simulink library "pmm"  (R2021b)
settings: Solver=VariableStepAuto  StartTime=0.0  StopTime=10.0  RelTol=1e-3
undefined symbols (not defined in the file or in its folder): ENUM_ACMAINRLYSTS_OPEN, ENUM_ACPRECHRGRLYSTS_OPEN, ENUM_B2VRLYSTA_OPEN, ENUM_BMSHVSTS_HVOPEN, ENUM_BRAKEPEDAL_RELEASED, ENUM_CACRLYDEM_CLOSE, ENUM_CACRLYSTS_OPEN, ENUM_CHRGFAULT_ACRLYFAIL, ENUM_CHRGFAULT_BCUHVFAIL, ENUM_CHRGFAULT_BCUNEGFAIL, ENUM_CHRGFAULT_BCUTIMEOUT, ENUM_CHRGFAULT_DCDCENABLE, ENUM_CHRGFAULT_DCDCRLYFAIL, ENUM_CHRGFAULT_HVILFAIL, ENUM_CHRGFAULT_PDUHVFAIL, ENUM_CHRGFAULT_RLYCHKFAIL, ENUM_DCDCEACPCURLYSTA_CLOSED, ENUM_DCDCEACPCURLYSTA_FAILTOCLOSE, ENUM_DCDCEACPCURLYSTA_OPEN, ENUM_DCDCEACPCURLYSTA_WELDED, ENUM_DCDCENABLESTS_READY, ENUM_DCDCRLYSTS_OPEN, ENUM_EHPSRLYDEM_CLOSE, ENUM_EHPSRLYSTS_OPEN, ENUM_FOGRLYENCMD_DISABLE, ENUM_GEARACTUALPOSN_D, ENUM_HVPWROFFREQ_POWEROFF, ENUM_KEYSTATUS_OFF, ENUM_KEYSTATUS_ON, ENUM_KEYSTATUS_START, ENUM_LOWBATTVOLTAGE_NORMAL, ENUM_LOWBATTVOLTAGE_POWERDOWN, ENUM_LOWBATTVOLTAGE_POWERUP, ENUM_MCUHVLOOP_POWEROFF, ENUM_MCUHVLOOPSTS_OPEN, ENUM_MCUMAINRLYSTS_OPEN, ENUM_MCUPRECHRGRLYSTS_OPEN, ENUM_PDFAULT_ACRLYOPEN, ENUM_PDFAULT_BCUDISABLE, ENUM_PDFAULT_DCDCDISABLE, ENUM_PDFAULT_DCDCRLYOPEN, ENUM_PDFAULT_EACDISABLE, ENUM_PDFAULT_EACRLYOPEN, ENUM_PDFAULT_EHPSDISABLE, ENUM_PDFAULT_EHPSRLYOPEN, ENUM_PDFAULT_MCUDISABLE, ENUM_PDFAULT_MCUDISCHRG, ENUM_PDFAULT_MCURLYOPEN, ENUM_PEUSELFCHKSTS_NOFAULT, ENUM_PLUGINSTS_NOPLUGIN, ENUM_PLUGINSTS_PLUGIN, ENUM_PMMMODE_DRIVE, ENUM_PMMMODE_LVBATCHRG, ENUM_PUSTATE_DCDCENABLE, ENUM_PUSTATE_EACPRESCHECK, ENUM_PUSTATE_EHPSENABLE, ENUM_PUSTATE_MCUENABLE, ENUM_PUSTATE_PDUMCURLYCLOSED, ENUM_PUSTATE_POWERUPFAIL, ENUM_TARGETGEAR_REVERSE ... (+126)
libraries: hcu_lib x45, simulink x5, ddm x1, dsc x1
(part 5 of 7)

== system pmm/PMM/PowerModeManagement/PMM State Change Configuration/PMM Initialize to PowerUp State ==
  note: [(VPMM_HVSelfChkCompleted4PU_flg
      | && VPSA_Keystatus_enum == ENUM_KEYSTATUS_START
      | && VINP_DCChrgConnectSts_enum == ENUM_PLUGINSTS_NOPLUGIN)
      |
      | || (!VSCP_LVchrgSvrMode_flg
      | && VPMM_LVChrgPreActFinished_flg
      | && VINP_ParkBrakeSW_flg
      | && VINP_B2VSOC_pct > KPMM_LVChrgEnHVSOC_pct)
      |
      | && (!VPMM_HVILEmergencyStop_flg)]
  VPSA_Keystatus_enum : Inport
  VINP_DCChrgConnectSts_enum : Inport  Port=2
  VPMM_HVILEmergencyStop_flg : Inport  Port=3
  VDMM_ProhibitPowerUp_flg : Inport  Port=4
  VSCP_LVchrgSvrMode_flg : Inport  Port=5
  VPMM_LVChrgPreActFinished_flg : Inport  Port=6
  VINP_ParkBrakeSW_flg : Inport  Port=7
  VINP_B2VSOC_pct : Inport  Port=8
  AND : Logic  Inputs=4  AllPortsSameDT=off  OutDataTypeStr=boolean
  AND1 : Logic  Inputs=5  AllPortsSameDT=off  OutDataTypeStr=boolean
  Constant2 : Constant  Value=ENUM_KEYSTATUS_START
  Constant3 : Constant  Value=ENUM_PLUGINSTS_NOPLUGIN
  Equal : RelationalOperator  Operator===  OutDataTypeStr=boolean  RndMeth=Simplest
  Equal1 : RelationalOperator  Operator===  OutDataTypeStr=boolean  RndMeth=Simplest
  NOT{,1..3} (4 alike) : Logic  Operator=NOT  AllPortsSameDT=off  OutDataTypeStr=boolean
  OR : Logic  Operator=OR  AllPortsSameDT=off  OutDataTypeStr=boolean
  Relay : Relay  OnSwitchValue=KPMM_LVChrgEnHVSOC_pct  OffSwitchValue=KPMM_LVChrgDisHVSOC_pct  OnOutputValue=TRUE  OffOutputValue=FALSE  OutDataTypeStr=boolean
  VPMM_Initialize2PowerUp_flg : Outport
  VPMM_LVChrgInit2PowerUp_flg : Outport  Port=2
  wires:
  NOT1/1 -> AND/4
  [VDMM_ProhibitPowerUp_flg] -> NOT1/1
  [VPSA_Keystatus_enum] -> Equal/1
  Constant2/1 -> Equal/2
  [VPMM_HVILEmergencyStop_flg] -> NOT/1
  VINP_DCChrgConnectSts_enum/1 -> [VINP_DCChrgConnectSts_enum]
  VPMM_HVILEmergencyStop_flg/1 -> [VPMM_HVILEmergencyStop_flg]
  VPSA_Keystatus_enum/1 -> [VPSA_Keystatus_enum]
  [VINP_DCChrgConnectSts_enum] -> Equal1/1
  Constant3/1 -> Equal1/2
  Equal/1 -> AND/1
  Equal1/1 -> AND/2
  NOT/1 -> AND/3
  VDMM_ProhibitPowerUp_flg/1 -> [VDMM_ProhibitPowerUp_flg]
  AND/1 -> OR/1
  OR/1 -> VPMM_Initialize2PowerUp_flg/1  "VPMM_Initialize2PowerUp_flg"
  NOT2/1 -> AND1/1
  [VSCP_LVchrgSvrMode_flg] -> NOT2/1
  [VPMM_LVChrgPreActFinished_flg] -> AND1/2
  [VINP_ParkBrakeSW_flg] -> AND1/3
  [VINP_B2VSOC_pct] -> Relay/1
  Relay/1 -> AND1/4
  AND1/1 -> OR/2, VPMM_LVChrgInit2PowerUp_flg/1  "VPMM_LVChrgInit2PowerUp_flg"
  VSCP_LVchrgSvrMode_flg/1 -> [VSCP_LVchrgSvrMode_flg]
  VPMM_LVChrgPreActFinished_flg/1 -> [VPMM_LVChrgPreActFinished_flg]
  VINP_ParkBrakeSW_flg/1 -> [VINP_ParkBrakeSW_flg]
  VINP_B2VSOC_pct/1 -> [VINP_B2VSOC_pct]
  NOT3/1 -> AND1/5
  [VPMM_HVILEmergencyStop_flg] -> NOT3/1

== system pmm/PMM/PowerModeManagement/PMM State Change Configuration/PMM PowerUp to PowerDown State ==
  note: [VPSA_Keystatus_enum == ENUM_KEYSTATUS_OFF || VPSA_EmergencyShutDown_flg ||
      | VPMM_HVILEmergencyStop_flg ||
      | VPMM_LostCom_flg ||
      | VPMM_RCIncorrect_flg ||
      | VDMM_VCUPowerVolHigh_flg ||
      | VDMM_VCUPowerVolLow_flg ||...
      | VDMM_WireFailure_flg]
  VPSA_Keystatus_enum : Inport
  VPSA_EmergencyShutDown_flg : Inport  Port=2
  VPMM_HVILEmergencyStop_flg : Inport  Port=3
  VPMM_LostCom_flg : Inport  Port=4
  VPMM_RCIncorrect_flg : Inport  Port=5
  VDMM_DCTVCUPowerVolHigh_flg : Inport  Port=6
  VDMM_DTCVCUPowerVolLow_flg : Inport  Port=7
  VDMM_DTCHVILWireFailure_flg : Inport  Port=8
  VDMM_NoFeedBack_flg : Inport  Port=9
  VDMM_WireFailure_flg : Inport  Port=10
  VPMM_LVChrgPreActFinished_flg : Inport  Port=11
  VPMM_PowerUpState_enum : Inport  Port=12
  VINP_B2VSOC_pct : Inport  Port=13
  VINP_ParkBrakeSW_flg : Inport  Port=14
  AND : Logic  AllPortsSameDT=off  OutDataTypeStr=boolean
  Constant : Constant  Value=ENUM_PUSTATE_POWERUPFAIL
  Constant2 : Constant  Value=ENUM_KEYSTATUS_OFF
  Equal : RelationalOperator  Operator===  OutDataTypeStr=boolean  RndMeth=Simplest
  Equal1 : RelationalOperator  Operator===  OutDataTypeStr=boolean  RndMeth=Simplest
  NOT : Logic  Operator=NOT  AllPortsSameDT=off  OutDataTypeStr=boolean
  NOT1 : Logic  Operator=NOT  AllPortsSameDT=off  OutDataTypeStr=boolean
  OR : Logic  Operator=OR  Inputs=11  AllPortsSameDT=off  OutDataTypeStr=boolean
  OR1 : Logic  Operator=OR  Inputs=3  AllPortsSameDT=off  OutDataTypeStr=boolean
  Relay : Relay  OnSwitchValue=KPMM_LVChrgEnHVSOC_pct  OffSwitchValue=KPMM_LVChrgDisHVSOC_pct  OnOutputValue=TRUE  OffOutputValue=FALSE  OutDataTypeStr=boolean
  VPMM_PowerUp2PowerDown_flg : Outport
  wires:
  VPMM_LostCom_flg/1 -> [VPMM_LostCom_flg]
  VPSA_Keystatus_enum/1 -> [VPSA_Keystatus_enum]
  [VPMM_HVILEmergencyStop_flg] -> OR/3
  VPSA_EmergencyShutDown_flg/1 -> [VPSA_EmergencyShutDown_flg]
  [VPMM_LostCom_flg] -> OR/4
  Constant2/1 -> Equal/2
  [VPSA_EmergencyShutDown_flg] -> OR/2
  Equal/1 -> OR/1
  [VPSA_Keystatus_enum] -> Equal/1
  VPMM_HVILEmergencyStop_flg/1 -> [VPMM_HVILEmergencyStop_flg]
  OR/1 -> VPMM_PowerUp2PowerDown_flg/1  "VPMM_PowerUp2PowerDown_flg"
  [VPMM_RCIncorrect_flg] -> OR/5
  VPMM_RCIncorrect_flg/1 -> [VPMM_RCIncorrect_flg]
  VDMM_DCTVCUPowerVolHigh_flg/1 -> [VDMM_DTCVCUPowerVolHigh_flg]
  VDMM_DTCVCUPowerVolLow_flg/1 -> [VDMM_DTCVCUPowerVolLow_flg]
  [VDMM_DTCVCUPowerVolHigh_flg] -> OR/6
  [VDMM_DTCVCUPowerVolLow_flg] -> OR/7
  VDMM_DTCHVILWireFailure_flg/1 -> [VDMM_DTCHVILWireFailure_flg]
  [VDMM_DTCHVILWireFailure_flg] -> OR/8
  VDMM_NoFeedBack_flg/1 -> [VDMM_NoFeedBack_flg]
  [VDMM_NoFeedBack_flg] -> OR/9
  VDMM_WireFailure_flg/1 -> [VDMM_WireFailure_flg]
  [VDMM_WireFailure_flg] -> OR/10
  VPMM_LVChrgPreActFinished_flg/1 -> [VPMM_LVChrgPreActFinished_flg]
  VPMM_PowerUpState_enum/1 -> [VPMM_PowerUpState_enum]
  [VPMM_PowerUpState_enum] -> Equal1/1
  Constant/1 -> Equal1/2
  [VPMM_LVChrgPreActFinished_flg] -> AND/1
  AND/1 -> OR/11
  Equal1/1 -> OR1/1
  [VINP_B2VSOC_pct] -> Relay/1
  NOT/1 -> OR1/3
  [VINP_ParkBrakeSW_flg] -> NOT/1
  OR1/1 -> AND/2
  VINP_B2VSOC_pct/1 -> [VINP_B2VSOC_pct]
  VINP_ParkBrakeSW_flg/1 -> [VINP_ParkBrakeSW_flg]
  Relay/1 -> NOT1/1
  NOT1/1 -> OR1/2

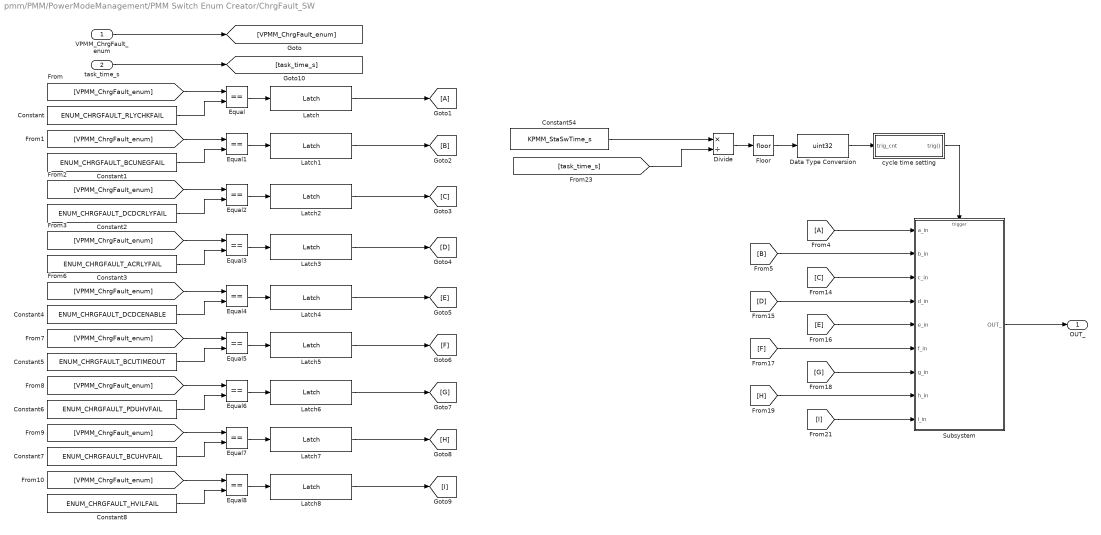
== system pmm/PMM/PowerModeManagement/PMM Switch Enum Creator/ChrgFault_SW ==
  VPMM_ChrgFault_enum : Inport
  task_time_s : Inport  Port=2
  Constant : Constant  Value=ENUM_CHRGFAULT_RLYCHKFAIL
  Constant1 : Constant  Value=ENUM_CHRGFAULT_BCUNEGFAIL
  Constant2 : Constant  Value=ENUM_CHRGFAULT_DCDCRLYFAIL
  Constant3 : Constant  Value=ENUM_CHRGFAULT_ACRLYFAIL
  Constant4 : Constant  Value=ENUM_CHRGFAULT_DCDCENABLE
  Constant5 : Constant  Value=ENUM_CHRGFAULT_BCUTIMEOUT
  Constant54 : Constant  Value=KPMM_StaSwTime_s
  Constant6 : Constant  Value=ENUM_CHRGFAULT_PDUHVFAIL
  Constant7 : Constant  Value=ENUM_CHRGFAULT_BCUHVFAIL
  Constant8 : Constant  Value=ENUM_CHRGFAULT_HVILFAIL
  Data Type Conversion : DataTypeConversion  OutDataTypeStr=uint32
  Divide : Product  Inputs=*/
  Equal{,1..8} (9 alike) : RelationalOperator  Operator===  OutDataTypeStr=boolean  RndMeth=Simplest
  Floor : Rounding
  Latch{,1..8} (9 alike) : hcu_lib/Basic_Blocks/Latch
      settings: SourceProductName=HCU Relative Block Library
  Subsystem : Subsystem
  cycle time setting : Stateflow chart  TreatAsAtomicUnit=on
  OUT_ : Outport
  wires:
  Constant54/1 -> Divide/1
  Divide/1 -> Floor/1
  [task_time_s] -> Divide/2
  Floor/1 -> Data Type Conversion/1
  task_time_s/1 -> [task_time_s]
  Subsystem/1(OUT_) -> OUT_/1
  [I] -> Subsystem/9(i_in)
  [H] -> Subsystem/8(h_in)
  [G] -> Subsystem/7(g_in)
  [F] -> Subsystem/6(f_in)
  [E] -> Subsystem/5(e_in)
  [D] -> Subsystem/4(d_in)
  [C] -> Subsystem/3(c_in)
  [B] -> Subsystem/2(b_in)
  [A] -> Subsystem/1(a_in)
  VPMM_ChrgFault_enum/1 -> [VPMM_ChrgFault_enum]
  [VPMM_ChrgFault_enum] -> Equal/1
  Constant/1 -> Equal/2
  Equal/1 -> Latch/1
  Equal1/1 -> Latch1/1
  Constant1/1 -> Equal1/2
  [VPMM_ChrgFault_enum] -> Equal1/1
  [VPMM_ChrgFault_enum] -> Equal2/1
  Constant2/1 -> Equal2/2
  Equal2/1 -> Latch2/1
  Equal3/1 -> Latch3/1
  Constant3/1 -> Equal3/2
  [VPMM_ChrgFault_enum] -> Equal3/1
  [VPMM_ChrgFault_enum] -> Equal4/1
  Constant4/1 -> Equal4/2
  Equal4/1 -> Latch4/1
  Equal5/1 -> Latch5/1
  Constant5/1 -> Equal5/2
  [VPMM_ChrgFault_enum] -> Equal5/1
  [VPMM_ChrgFault_enum] -> Equal6/1
  Constant6/1 -> Equal6/2
  Equal6/1 -> Latch6/1
  Equal7/1 -> Latch7/1
  Constant7/1 -> Equal7/2
  [VPMM_ChrgFault_enum] -> Equal7/1
  [VPMM_ChrgFault_enum] -> Equal8/1
  Constant8/1 -> Equal8/2
  Equal8/1 -> Latch8/1
  Latch/1 -> [A]
  Latch1/1 -> [B]
  Latch2/1 -> [C]
  Latch5/1 -> [F]
  Latch4/1 -> [E]
  Latch3/1 -> [D]
  Latch8/1 -> [I]
  Latch7/1 -> [H]
  Latch6/1 -> [G]
  Data Type Conversion/1 -> cycle time setting/1(trig_cnt)
  cycle time setting/1(trig()) -> Subsystem/Trigger

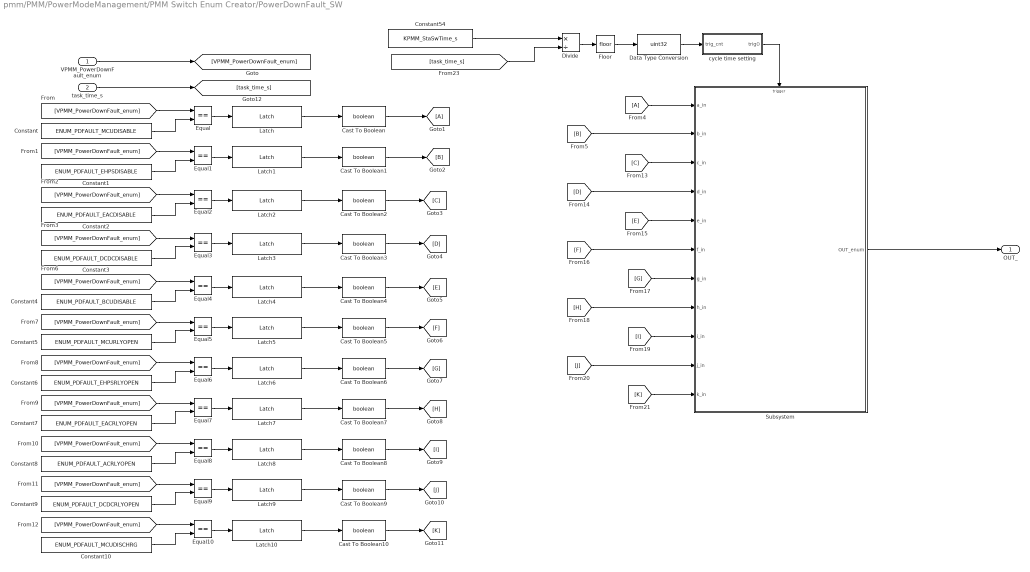
== system pmm/PMM/PowerModeManagement/PMM Switch Enum Creator/PowerDownFault_SW ==
  VPMM_PowerDownFault_enum : Inport
  task_time_s : Inport  Port=2
  Cast To Boolean{,1..10} (11 alike) : DataTypeConversion  OutDataTypeStr=boolean
  Constant : Constant  Value=ENUM_PDFAULT_MCUDISABLE
  Constant1 : Constant  Value=ENUM_PDFAULT_EHPSDISABLE
  Constant10 : Constant  Value=ENUM_PDFAULT_MCUDISCHRG
  Constant2 : Constant  Value=ENUM_PDFAULT_EACDISABLE
  Constant3 : Constant  Value=ENUM_PDFAULT_DCDCDISABLE
  Constant4 : Constant  Value=ENUM_PDFAULT_BCUDISABLE
  Constant5 : Constant  Value=ENUM_PDFAULT_MCURLYOPEN
  Constant54 : Constant  Value=KPMM_StaSwTime_s
  Constant6 : Constant  Value=ENUM_PDFAULT_EHPSRLYOPEN
  Constant7 : Constant  Value=ENUM_PDFAULT_EACRLYOPEN
  Constant8 : Constant  Value=ENUM_PDFAULT_ACRLYOPEN
  Constant9 : Constant  Value=ENUM_PDFAULT_DCDCRLYOPEN
  Data Type Conversion : DataTypeConversion  OutDataTypeStr=uint32
  Divide : Product  Inputs=*/
  Equal{,1..10} (11 alike) : RelationalOperator  Operator===  OutDataTypeStr=boolean  RndMeth=Simplest
  Floor : Rounding
  Latch{,1..10} (11 alike) : hcu_lib/Basic_Blocks/Latch
      settings: SourceProductName=HCU Relative Block Library
  Subsystem : Subsystem
  cycle time setting : Stateflow chart  TreatAsAtomicUnit=on
  OUT_ : Outport
  wires:
  VPMM_PowerDownFault_enum/1 -> [VPMM_PowerDownFault_enum]
  cycle time setting/1(trig()) -> Subsystem/Trigger
  task_time_s/1 -> [task_time_s]
  Constant54/1 -> Divide/1
  Divide/1 -> Floor/1
  [task_time_s] -> Divide/2
  Floor/1 -> Data Type Conversion/1
  [K] -> Subsystem/11(k_in)
  [J] -> Subsystem/10(j_in)
  [I] -> Subsystem/9(i_in)
  [H] -> Subsystem/8(h_in)
  [G] -> Subsystem/7(g_in)
  [F] -> Subsystem/6(f_in)
  [E] -> Subsystem/5(e_in)
  [D] -> Subsystem/4(d_in)
  [C] -> Subsystem/3(c_in)
  [B] -> Subsystem/2(b_in)
  [A] -> Subsystem/1(a_in)
  Subsystem/1(OUT_enum) -> OUT_/1
  Latch6/1 -> Cast To Boolean6/1
  Latch7/1 -> Cast To Boolean7/1
  Latch10/1 -> Cast To Boolean10/1
  Latch9/1 -> Cast To Boolean9/1
  Latch8/1 -> Cast To Boolean8/1
  Latch3/1 -> Cast To Boolean3/1
  Latch4/1 -> Cast To Boolean4/1
  Latch5/1 -> Cast To Boolean5/1
  Latch2/1 -> Cast To Boolean2/1
  Latch1/1 -> Cast To Boolean1/1
  Latch/1 -> Cast To Boolean/1
  Equal10/1 -> Latch10/1
  Constant10/1 -> Equal10/2
  [VPMM_PowerDownFault_enum] -> Equal10/1
  [VPMM_PowerDownFault_enum] -> Equal9/1
  Constant9/1 -> Equal9/2
  Equal9/1 -> Latch9/1
  Equal8/1 -> Latch8/1
  Constant8/1 -> Equal8/2
  [VPMM_PowerDownFault_enum] -> Equal8/1
  [VPMM_PowerDownFault_enum] -> Equal7/1
  Constant7/1 -> Equal7/2
  Equal7/1 -> Latch7/1
  Equal6/1 -> Latch6/1
  Constant6/1 -> Equal6/2
  [VPMM_PowerDownFault_enum] -> Equal6/1
  [VPMM_PowerDownFault_enum] -> Equal5/1
  Constant5/1 -> Equal5/2
  Equal5/1 -> Latch5/1
  Equal4/1 -> Latch4/1
  Constant4/1 -> Equal4/2
  [VPMM_PowerDownFault_enum] -> Equal4/1
  [VPMM_PowerDownFault_enum] -> Equal3/1
  Constant3/1 -> Equal3/2
  Equal3/1 -> Latch3/1
  Equal2/1 -> Latch2/1
  Constant2/1 -> Equal2/2
  [VPMM_PowerDownFault_enum] -> Equal2/1
  [VPMM_PowerDownFault_enum] -> Equal1/1
  Constant1/1 -> Equal1/2
  Equal1/1 -> Latch1/1
  Equal/1 -> Latch/1
  Constant/1 -> Equal/2
  [VPMM_PowerDownFault_enum] -> Equal/1
  Cast To Boolean/1 -> [A]
  Cast To Boolean1/1 -> [B]
  Cast To Boolean2/1 -> [C]
  Cast To Boolean3/1 -> [D]
  Cast To Boolean4/1 -> [E]
  Cast To Boolean5/1 -> [F]
  Cast To Boolean6/1 -> [G]
  Cast To Boolean7/1 -> [H]
  Cast To Boolean8/1 -> [I]
  Cast To Boolean9/1 -> [J]
  Cast To Boolean10/1 -> [K]
  Data Type Conversion/1 -> cycle time setting/1(trig_cnt)

== system pmm/PMM/PowerModeManagement/PMM Switch Enum Creator/PowerUpState_SW ==
  Sys_in : Inport
  a_in : Inport  Port=2
  b_in : Inport  Port=3
  c_in : Inport  Port=4
  d_in : Inport  Port=5
  e_in : Inport  Port=6
  a_enum : Inport  Port=7
  b_enum : Inport  Port=8
  c_enum : Inport  Port=9
  d_enum : Inport  Port=10
  e_enum : Inport  Port=11
  function : TriggerPort  TriggerType=function-call  VariantControl=Variant
  PowerUpState_SW : Stateflow chart  TreatAsAtomicUnit=on
  OUT_enum : Outport
  wires:
  Sys_in/1 -> PowerUpState_SW/1(Sys_in)
  PowerUpState_SW/1(OUT_enum) -> OUT_enum/1
  e_enum/1 -> PowerUpState_SW/11(e_enum)
  d_in/1 -> PowerUpState_SW/5(d_in)
  b_in/1 -> PowerUpState_SW/3(b_in)
  a_enum/1 -> PowerUpState_SW/7(a_enum)
  e_in/1 -> PowerUpState_SW/6(e_in)
  c_in/1 -> PowerUpState_SW/4(c_in)
  a_in/1 -> PowerUpState_SW/2(a_in)
  c_enum/1 -> PowerUpState_SW/9(c_enum)
  d_enum/1 -> PowerUpState_SW/10(d_enum)
  b_enum/1 -> PowerUpState_SW/8(b_enum)

== system pmm/PMM/PowerModeManagement/PMM Flag Creator /HVIL Judgement/Signal reach time counter ==
  signal_in : Inport
  time_step : Inport  Port=2
  time_reach : Inport  Port=3
  cnt_reset : Inport  Port=4
  cnt_max : Inport  Port=5
  cnt_min : Inport  Port=6
  Add : Sum
  Add1 : Sum  Inputs=+-
  Add2 : Sum
  Constant1 : Constant  Value=0
  Constant2 : Constant  OutDataTypeStr=single
  Constant3 : Constant  Value=0  OutDataTypeStr=single
  Logical Operator : Logic  Operator=NOT  AllPortsSameDT=off  OutDataTypeStr=boolean
  Logical Operator1 : Logic  AllPortsSameDT=off  OutDataTypeStr=boolean
  Max : MinMax  Function=max  Inputs=2
  Min : MinMax  Inputs=2
  Relational Operator : RelationalOperator  OutDataTypeStr=boolean  RndMeth=Simplest
  Switch : Switch  Criteria=u2 > Threshold
      settings: AttributesFormatString=%<Criteria>
  Switch1 : Switch  Criteria=u2 > Threshold
      settings: AttributesFormatString=%<Criteria>
  Switch2 : Switch  Criteria=u2 > Threshold
      settings: AttributesFormatString=%<Criteria>
  Unit Delay : UnitDelay  SampleTime=-1  HasFrameUpgradeWarning=on
  Unit Delay1 : UnitDelay  SampleTime=-1  HasFrameUpgradeWarning=on
  Unit Delay2 : UnitDelay  SampleTime=-1  HasFrameUpgradeWarning=on
  cnt_times : Outport
  wires:
  Min/1 -> cnt_times/1
  cnt_max/1 -> Min/2
  Max/1 -> Min/1
  cnt_min/1 -> Max/2
  Constant3/1 -> Switch2/1
  cnt_reset/1 -> Switch2/2
  Switch2/1 -> Unit Delay1/1, Max/1
  Switch/1 -> Switch2/3
  [cont_reset] -> Logical Operator1/2
  signal_in/1 -> Logical Operator1/1
  Logical Operator1/1 -> Switch1/2
  Logical Operator/1 -> [cont_reset]
  [cnt_flg] -> Switch/2
  Unit Delay2/1 -> Logical Operator/1
  Relational Operator/1 -> Unit Delay2/1, [cnt_flg]
  Add2/1 -> Switch/1
  Constant2/1 -> Add2/1
  Unit Delay1/1 -> Add2/2, Switch/3
  time_step/1 -> Add1/2, Add/1
  Unit Delay/1 -> Add/2
  Switch1/1 -> Unit Delay/1, Relational Operator/1
  Add/1 -> Switch1/1
  Constant1/1 -> Switch1/3
  time_reach/1 -> Add1/1
  Add1/1 -> Relational Operator/2

== system pmm/PMM/PowerModeManagement/PMM Flag Creator /HVIL Judgement/Signal reach time counter1 ==
  signal_in : Inport
  time_step : Inport  Port=2
  time_reach : Inport  Port=3
  cnt_reset : Inport  Port=4
  cnt_max : Inport  Port=5
  cnt_min : Inport  Port=6
  Add : Sum
  Add1 : Sum  Inputs=+-
  Add2 : Sum
  Constant1 : Constant  Value=0
  Constant2 : Constant  OutDataTypeStr=single
  Constant3 : Constant  Value=0  OutDataTypeStr=single
  Logical Operator : Logic  Operator=NOT  AllPortsSameDT=off  OutDataTypeStr=boolean
  Logical Operator1 : Logic  AllPortsSameDT=off  OutDataTypeStr=boolean
  Max : MinMax  Function=max  Inputs=2
  Min : MinMax  Inputs=2
  Relational Operator : RelationalOperator  OutDataTypeStr=boolean  RndMeth=Simplest
  Switch : Switch  Criteria=u2 > Threshold
      settings: AttributesFormatString=%<Criteria>
  Switch1 : Switch  Criteria=u2 > Threshold
      settings: AttributesFormatString=%<Criteria>
  Switch2 : Switch  Criteria=u2 > Threshold
      settings: AttributesFormatString=%<Criteria>
  Unit Delay : UnitDelay  SampleTime=-1  HasFrameUpgradeWarning=on
  Unit Delay1 : UnitDelay  SampleTime=-1  HasFrameUpgradeWarning=on
  Unit Delay2 : UnitDelay  SampleTime=-1  HasFrameUpgradeWarning=on
  cnt_times : Outport
  wires:
  Add1/1 -> Relational Operator/2
  time_reach/1 -> Add1/1
  Constant1/1 -> Switch1/3
  Add/1 -> Switch1/1
  Switch1/1 -> Relational Operator/1, Unit Delay/1
  Unit Delay/1 -> Add/2
  time_step/1 -> Add/1, Add1/2
  Unit Delay1/1 -> Switch/3, Add2/2
  Constant2/1 -> Add2/1
  Add2/1 -> Switch/1
  Relational Operator/1 -> [cnt_flg], Unit Delay2/1
  Unit Delay2/1 -> Logical Operator/1
  [cnt_flg] -> Switch/2
  Logical Operator/1 -> [cont_reset]
  Logical Operator1/1 -> Switch1/2
  signal_in/1 -> Logical Operator1/1
  [cont_reset] -> Logical Operator1/2
  Switch/1 -> Switch2/3
  Switch2/1 -> Max/1, Unit Delay1/1
  cnt_reset/1 -> Switch2/2
  Constant3/1 -> Switch2/1
  cnt_min/1 -> Max/2
  Max/1 -> Min/1
  cnt_max/1 -> Min/2
  Min/1 -> cnt_times/1

== system pmm/PMM/PowerModeManagement/PMM Flag Creator /Low Battery Voltage/Long Idle Flasher ==
  task_time_s1 : Inport
  Constant10 : Constant  Value=KPMM_LongIdleBuzzerOFF_s  VectorParams1D=off
  Constant11 : Constant  Value=KPMM_LongIdleBuzzerFlash_cnt  VectorParams1D=off
  Constant12 : Constant  Value=KPMM_LongIdleBuzzerWait_s  VectorParams1D=off
  Constant22 : Constant  Value=KPMM_LongIdleBuzzerON_s  VectorParams1D=off
  Data Type Conversion3 : DataTypeConversion  OutDataTypeStr=boolean
  Reverse Buzzer Flasher : Subsystem
  VPMM_LongIdleBuzzer_flg : Outport
  wires:
  Reverse Buzzer Flasher/1(SigOut) -> Data Type Conversion3/1
  Data Type Conversion3/1 -> VPMM_LongIdleBuzzer_flg/1  "VPMM_LongIdleBuzzer_flg"
  task_time_s1/1 -> [task_time_s]
  Constant12/1 -> Reverse Buzzer Flasher/5(Wait_s)
  Constant22/1 -> Reverse Buzzer Flasher/2(ON_s)
  Constant11/1 -> Reverse Buzzer Flasher/4(Cycle_cnt)
  Constant10/1 -> Reverse Buzzer Flasher/3(OFF_s)
  [task_time_s] -> Reverse Buzzer Flasher/1(Task_Time_s)

== system pmm/PMM/PowerModeManagement/PMM Flag Creator /Low Battery Voltage/Low Voltage Charge Action Flasher ==
  task_time_s : Inport
  Brake Lamp  Flasher : Subsystem
  Constant : Constant  Value=FALSE
  Constant10 : Constant  Value=KPMM_LVChrgDuBrkLampON_s
  Constant11 : Constant  Value=KPMM_LVChrgDuBrkLampOFF_s  VectorParams1D=off
  Constant12 : Constant  Value=KPMM_LVChrgDuBrkLampFlash_cnt  VectorParams1D=off
  Constant13 : Constant  Value=KPMM_LVChrgDuBrkLampWait_s  VectorParams1D=off
  Constant22 : Constant  Value=KPMM_LVChrgDuRBuzzerON_s  VectorParams1D=off
  Constant3 : Constant  Value=KPMM_LVChrgDuRBuzzerOFF_s  VectorParams1D=off
  Constant4 : Constant  Value=KPMM_LVChrgDuRBuzzerFlash_cnt  VectorParams1D=off
  Constant5 : Constant  Value=KPMM_LVChrgDuRBuzzerWait_s  VectorParams1D=off
  Data Type Conversion : DataTypeConversion  OutDataTypeStr=boolean
  Data Type Conversion2 : DataTypeConversion  OutDataTypeStr=boolean
  Reverse Buzzer Flasher : Subsystem
  VPMM_LVChrgDuRBuzzer_flg : Outport
  VPMM_LVChrgDuRLamp_flg : Outport  Port=2
  VPMM_LVChrgDuBrkLamp_flg : Outport  Port=3
  wires:
  Data Type Conversion2/1 -> VPMM_LVChrgDuBrkLamp_flg/1  "VPMM_LVChrgDuBrkLamp_flg"
  Brake Lamp  Flasher/1(SigOut) -> Data Type Conversion2/1
  Reverse Buzzer Flasher/1(SigOut) -> Data Type Conversion/1
  Data Type Conversion/1 -> VPMM_LVChrgDuRBuzzer_flg/1  "VPMM_LVChrgDuRBuzzer_flg"
  task_time_s/1 -> [task_time_s]
  Constant4/1 -> Reverse Buzzer Flasher/4(Cycle_cnt)
  Constant10/1 -> Brake Lamp  Flasher/2(ON_s)
  Constant5/1 -> Reverse Buzzer Flasher/5(Wait_s)
  Constant13/1 -> Brake Lamp  Flasher/5(Wait_s)
  Constant11/1 -> Brake Lamp  Flasher/3(OFF_s)
  Constant12/1 -> Brake Lamp  Flasher/4(Cycle_cnt)
  [task_time_s] -> Brake Lamp  Flasher/1(Task_Time_s)
  Constant22/1 -> Reverse Buzzer Flasher/2(ON_s)
  Constant3/1 -> Reverse Buzzer Flasher/3(OFF_s)
  [task_time_s] -> Reverse Buzzer Flasher/1(Task_Time_s)
  Constant/1 -> VPMM_LVChrgDuRLamp_flg/1  "VPMM_LVChrgDuRLamp_flg"

== system pmm/PMM/PowerModeManagement/PMM Flag Creator /Low Battery Voltage/Low Voltage Charge Pre-Action Flasher ==
  task_time_s : Inport
  Brake Lamp  Flasher : Subsystem
  Constant10 : Constant  Value=KPMM_LVChrgPreActBrkLampON_s  VectorParams1D=off
  Constant11 : Constant  Value=KPMM_LVChrgPreActBrkLampOFF_s  VectorParams1D=off
  Constant12 : Constant  Value=KPMM_LVChrgPreActBrkLampFlash_cnt  VectorParams1D=off
  Constant13 : Constant  Value=KPMM_LVChrgPreActBrkLampWait_s  VectorParams1D=off
  Constant22 : Constant  Value=KPMM_LVChrgPreActRBuzzerON_s  VectorParams1D=off
  Constant3 : Constant  Value=KPMM_LVChrgPreActRBuzzerOFF_s  VectorParams1D=off
  Constant4 : Constant  Value=KPMM_LVChrgPreActRBuzzerFlash_cnt  VectorParams1D=off
  Constant5 : Constant  Value=KPMM_LVChrgPreActRBuzzerWait_s  VectorParams1D=off
  Constant6 : Constant  Value=KPMM_LVChrgPreActRLampON_s  VectorParams1D=off
  Constant7 : Constant  Value=KPMM_LVChrgPreActRLampOFF_s  VectorParams1D=off
  Constant8 : Constant  Value=KPMM_LVChrgPreActRLampFlash_cnt  VectorParams1D=off
  Constant9 : Constant  Value=KPMM_LVChrgPreActRLampWait_s  VectorParams1D=off
  Data Type Conversion : DataTypeConversion  OutDataTypeStr=boolean
  Data Type Conversion1 : DataTypeConversion  OutDataTypeStr=boolean
  Data Type Conversion2 : DataTypeConversion  OutDataTypeStr=boolean
  Reverse Buzzer Flasher : Subsystem
  Reverse Lamp Flasher : Subsystem
  VPMM_LVChrgPreActRBuzzer_flg : Outport
  VPMM_LVChrgPreActRLamp_flg : Outport  Port=2
  VPMM_LVChrgPreActBrkLamp_flg : Outport  Port=3
  wires:
  [task_time_s] -> Reverse Buzzer Flasher/1(Task_Time_s)
  Constant7/1 -> Reverse Lamp Flasher/3(OFF_s)
  Constant6/1 -> Reverse Lamp Flasher/2(ON_s)
  Constant3/1 -> Reverse Buzzer Flasher/3(OFF_s)
  [task_time_s] -> Reverse Lamp Flasher/1(Task_Time_s)
  Constant9/1 -> Reverse Lamp Flasher/5(Wait_s)
  Constant22/1 -> Reverse Buzzer Flasher/2(ON_s)
  Constant8/1 -> Reverse Lamp Flasher/4(Cycle_cnt)
  [task_time_s] -> Brake Lamp  Flasher/1(Task_Time_s)
  Constant12/1 -> Brake Lamp  Flasher/4(Cycle_cnt)
  Constant11/1 -> Brake Lamp  Flasher/3(OFF_s)
  Constant13/1 -> Brake Lamp  Flasher/5(Wait_s)
  Constant5/1 -> Reverse Buzzer Flasher/5(Wait_s)
  Constant10/1 -> Brake Lamp  Flasher/2(ON_s)
  Constant4/1 -> Reverse Buzzer Flasher/4(Cycle_cnt)
  task_time_s/1 -> [task_time_s]
  Data Type Conversion/1 -> VPMM_LVChrgPreActRBuzzer_flg/1  "VPMM_LVChrgPreActRBuzzer_flg"
  Reverse Buzzer Flasher/1(SigOut) -> Data Type Conversion/1
  Reverse Lamp Flasher/1(SigOut) -> Data Type Conversion1/1
  Data Type Conversion1/1 -> VPMM_LVChrgPreActRLamp_flg/1  "VPMM_LVChrgPreActRLamp_flg"
  Brake Lamp  Flasher/1(SigOut) -> Data Type Conversion2/1
  Data Type Conversion2/1 -> VPMM_LVChrgPreActBrkLamp_flg/1  "VPMM_LVChrgPreActBrkLamp_flg"

== system pmm/PMM/PowerModeManagement/PMM Switch Enum Creator/ChrgFault_SW/Subsystem ==
  a_in : Inport
  b_in : Inport  Port=2
  c_in : Inport  Port=3
  d_in : Inport  Port=4
  e_in : Inport  Port=5
  f_in : Inport  Port=6
  g_in : Inport  Port=7
  h_in : Inport  Port=8
  i_in : Inport  Port=9
  function : TriggerPort  TriggerType=function-call  VariantControl=Variant
  Chart : Stateflow chart  TreatAsAtomicUnit=on
  Constant10 : Constant  Value=ENUM_CHRGFAULT_BCUNEGFAIL
  Constant11 : Constant  Value=ENUM_CHRGFAULT_DCDCRLYFAIL
  Constant12 : Constant  Value=ENUM_CHRGFAULT_ACRLYFAIL
  Constant13 : Constant  Value=ENUM_CHRGFAULT_DCDCENABLE
  Constant14 : Constant  Value=ENUM_CHRGFAULT_BCUTIMEOUT
  Constant15 : Constant  Value=ENUM_CHRGFAULT_PDUHVFAIL
  Constant16 : Constant  Value=ENUM_CHRGFAULT_BCUHVFAIL
  Constant17 : Constant  Value=ENUM_CHRGFAULT_HVILFAIL
  Constant9 : Constant  Value=ENUM_CHRGFAULT_RLYCHKFAIL
  OUT_ : Outport
  wires:
  e_in/1 -> Chart/5(e_in)
  g_in/1 -> Chart/7(g_in)
  a_in/1 -> Chart/1(a_in)
  f_in/1 -> Chart/6(f_in)
  h_in/1 -> Chart/8(h_in)
  Chart/1(OUT_) -> OUT_/1
  c_in/1 -> Chart/3(c_in)
  Constant17/1 -> Chart/18(i_enum)
  Constant15/1 -> Chart/16(g_enum)
  b_in/1 -> Chart/2(b_in)
  Constant13/1 -> Chart/14(e_enum)
  d_in/1 -> Chart/4(d_in)
  Constant10/1 -> Chart/11(b_enum)
  i_in/1 -> Chart/9(i_in)
  Constant11/1 -> Chart/12(c_enum)
  Constant12/1 -> Chart/13(d_enum)
  Constant16/1 -> Chart/17(h_enum)
  Constant9/1 -> Chart/10(a_enum)
  Constant14/1 -> Chart/15(f_enum)

== system pmm/PMM/PowerModeManagement/PMM Switch Enum Creator/PowerDownFault_SW/Subsystem ==
  a_in : Inport
  b_in : Inport  Port=2
  c_in : Inport  Port=3
  d_in : Inport  Port=4
  e_in : Inport  Port=5
  f_in : Inport  Port=6
  g_in : Inport  Port=7
  h_in : Inport  Port=8
  i_in : Inport  Port=9
  j_in : Inport  Port=10
  k_in : Inport  Port=11
  function : TriggerPort  TriggerType=function-call  VariantControl=Variant
  Chart : Stateflow chart  TreatAsAtomicUnit=on
  Constant11 : Constant  Value=ENUM_PDFAULT_MCUDISABLE
  Constant12 : Constant  Value=ENUM_PDFAULT_EHPSDISABLE
  Constant13 : Constant  Value=ENUM_PDFAULT_EACDISABLE
  Constant14 : Constant  Value=ENUM_PDFAULT_DCDCDISABLE
  Constant15 : Constant  Value=ENUM_PDFAULT_BCUDISABLE
  Constant16 : Constant  Value=ENUM_PDFAULT_MCURLYOPEN
  Constant17 : Constant  Value=ENUM_PDFAULT_EHPSRLYOPEN
  Constant18 : Constant  Value=ENUM_PDFAULT_EACRLYOPEN
  Constant19 : Constant  Value=ENUM_PDFAULT_ACRLYOPEN
  Constant20 : Constant  Value=ENUM_PDFAULT_DCDCRLYOPEN
  Constant21 : Constant  Value=ENUM_PDFAULT_MCUDISCHRG
  OUT_enum : Outport
  wires:
  j_in/1 -> Chart/10(j_in)
  h_in/1 -> Chart/8(h_in)
  f_in/1 -> Chart/6(f_in)
  d_in/1 -> Chart/4(d_in)
  b_in/1 -> Chart/2(b_in)
  Chart/1(OUT_enum) -> OUT_enum/1
  Constant19/1 -> Chart/20(i_enum)
  Constant21/1 -> Chart/22(k_enum)
  Constant17/1 -> Chart/18(g_enum)
  a_in/1 -> Chart/1(a_in)
  i_in/1 -> Chart/9(i_in)
  Constant13/1 -> Chart/14(c_enum)
  Constant18/1 -> Chart/19(h_enum)
  Constant11/1 -> Chart/12(a_enum)
  k_in/1 -> Chart/11(k_in)
  Constant15/1 -> Chart/16(e_enum)
  Constant12/1 -> Chart/13(b_enum)
  Constant14/1 -> Chart/15(d_enum)
  Constant20/1 -> Chart/21(j_enum)
  e_in/1 -> Chart/5(e_in)
  g_in/1 -> Chart/7(g_in)
  c_in/1 -> Chart/3(c_in)
  Constant16/1 -> Chart/17(f_enum)

== system pmm/PMM/PowerModeManagement/PMM Flag Creator /Low Battery Voltage/Long Idle Flasher/Reverse Buzzer Flasher ==
  Task_Time_s : Inport
  ON_s : Inport  Port=2
  OFF_s : Inport  Port=3
  Cycle_cnt : Inport  Port=4
  Wait_s : Inport  Port=5
  Add : Sum  Inputs=+-
  Chart : Stateflow chart  TreatAsAtomicUnit=on
  Constant4 : Constant  Value=ONE_INT
  Data Type Conversion{,1..3} (4 alike) : DataTypeConversion
  Divide : Product  Inputs=*/
  Divide1 : Product  Inputs=*/
  Divide2 : Product  Inputs=*/
  Floor : Rounding
  Floor1 : Rounding
  Floor2 : Rounding
  SigOut : Outport
  wires:
  Floor2/1 -> Data Type Conversion3/1  "WAIT_cnt"
  Floor1/1 -> Data Type Conversion2/1  "OFF_cnt"
  Divide/1 -> Floor/1
  Divide1/1 -> Floor1/1
  Add/1 -> Data Type Conversion1/1  "Cycle_cnt"
  Floor/1 -> Data Type Conversion/1  "ON_cnt"
  Divide2/1 -> Floor2/1
  Constant4/1 -> Add/2
  [Cycle_cnt] -> Add/1  "Cycle_cnt"
  ON_s/1 -> [ON_s]
  OFF_s/1 -> [OFF_s]
  [TaskTime_s] -> Divide/2
  [TaskTime_s] -> Divide2/2
  [Wait_s] -> Divide2/1  "Wait_s"
  [TaskTime_s] -> Divide1/2
  [ON_s] -> Divide/1  "ON_s"
  [OFF_s] -> Divide1/1  "OFF_s"
  Cycle_cnt/1 -> [Cycle_cnt]
  Wait_s/1 -> [Wait_s]
  Chart/1(out) -> SigOut/1
  Task_Time_s/1 -> [TaskTime_s]
  Data Type Conversion/1 -> Chart/1(ON_cnt)
  Data Type Conversion2/1 -> Chart/2(OFF_cnt)
  Data Type Conversion3/1 -> Chart/3(WAIT_cnt)
  Data Type Conversion1/1 -> Chart/4(Cycle_cnt)

== system pmm/PMM/PowerModeManagement/PMM Flag Creator /Low Battery Voltage/Low Voltage Charge Action Flasher/Brake Lamp  Flasher ==
  Task_Time_s : Inport
  ON_s : Inport  Port=2
  OFF_s : Inport  Port=3
  Cycle_cnt : Inport  Port=4
  Wait_s : Inport  Port=5
  Add : Sum  Inputs=+-
  Chart : Stateflow chart  TreatAsAtomicUnit=on
  Constant4 : Constant  Value=ONE_INT
  Data Type Conversion{,1..3} (4 alike) : DataTypeConversion
  Divide : Product  Inputs=*/
  Divide1 : Product  Inputs=*/
  Divide2 : Product  Inputs=*/
  Floor : Rounding
  Floor1 : Rounding
  Floor2 : Rounding
  SigOut : Outport
  wires:
  Divide/1 -> Floor/1
  Divide1/1 -> Floor1/1
  Divide2/1 -> Floor2/1
  Constant4/1 -> Add/2
  [Cycle_cnt] -> Add/1  "Cycle_cnt"
  ON_s/1 -> [ON_s]
  OFF_s/1 -> [OFF_s]
  [TaskTime_s] -> Divide/2
  [TaskTime_s] -> Divide2/2
  [Wait_s] -> Divide2/1  "Wait_s"
  [TaskTime_s] -> Divide1/2
  [ON_s] -> Divide/1  "ON_s"
  [OFF_s] -> Divide1/1  "OFF_s"
  Cycle_cnt/1 -> [Cycle_cnt]
  Wait_s/1 -> [Wait_s]
  Chart/1(out) -> SigOut/1
  Task_Time_s/1 -> [TaskTime_s]
  Data Type Conversion1/1 -> Chart/4(Cycle_cnt)
  Data Type Conversion2/1 -> Chart/2(OFF_cnt)
  Data Type Conversion3/1 -> Chart/3(WAIT_cnt)
  Floor1/1 -> Data Type Conversion2/1  "OFF_cnt"
  Floor/1 -> Data Type Conversion/1  "ON_cnt"
  Floor2/1 -> Data Type Conversion3/1  "WAIT_cnt"
  Add/1 -> Data Type Conversion1/1  "Cycle_cnt"
  Data Type Conversion/1 -> Chart/1(ON_cnt)

== system pmm/PMM/PowerModeManagement/PMM Flag Creator /Low Battery Voltage/Low Voltage Charge Action Flasher/Reverse Buzzer Flasher ==
  Task_Time_s : Inport
  ON_s : Inport  Port=2
  OFF_s : Inport  Port=3
  Cycle_cnt : Inport  Port=4
  Wait_s : Inport  Port=5
  Add : Sum  Inputs=+-
  Chart : Stateflow chart  TreatAsAtomicUnit=on
  Constant4 : Constant  Value=ONE_INT
  Data Type Conversion{,1..3} (4 alike) : DataTypeConversion
  Divide : Product  Inputs=*/
  Divide1 : Product  Inputs=*/
  Divide2 : Product  Inputs=*/
  Floor : Rounding
  Floor1 : Rounding
  Floor2 : Rounding
  SigOut : Outport
  wires:
  Divide/1 -> Floor/1
  Divide1/1 -> Floor1/1
  Divide2/1 -> Floor2/1
  Constant4/1 -> Add/2
  [Cycle_cnt] -> Add/1  "Cycle_cnt"
  ON_s/1 -> [ON_s]
  OFF_s/1 -> [OFF_s]
  [TaskTime_s] -> Divide/2
  [TaskTime_s] -> Divide2/2
  [Wait_s] -> Divide2/1  "Wait_s"
  [TaskTime_s] -> Divide1/2
  [ON_s] -> Divide/1  "ON_s"
  [OFF_s] -> Divide1/1  "OFF_s"
  Cycle_cnt/1 -> [Cycle_cnt]
  Wait_s/1 -> [Wait_s]
  Chart/1(out) -> SigOut/1
  Task_Time_s/1 -> [TaskTime_s]
  Data Type Conversion3/1 -> Chart/3(WAIT_cnt)
  Data Type Conversion/1 -> Chart/1(ON_cnt)
  Data Type Conversion1/1 -> Chart/4(Cycle_cnt)
  Data Type Conversion2/1 -> Chart/2(OFF_cnt)
  Floor/1 -> Data Type Conversion/1  "ON_cnt"
  Floor1/1 -> Data Type Conversion2/1  "OFF_cnt"
  Floor2/1 -> Data Type Conversion3/1  "WAIT_cnt"
  Add/1 -> Data Type Conversion1/1  "Cycle_cnt"

== system pmm/PMM/PowerModeManagement/PMM Flag Creator /Low Battery Voltage/Low Voltage Charge Pre-Action Flasher/Brake Lamp  Flasher ==
  Task_Time_s : Inport
  ON_s : Inport  Port=2
  OFF_s : Inport  Port=3
  Cycle_cnt : Inport  Port=4
  Wait_s : Inport  Port=5
  Add : Sum  Inputs=+-
  Chart : Stateflow chart  TreatAsAtomicUnit=on
  Constant4 : Constant  Value=ONE_INT
  Data Type Conversion{,1..3} (4 alike) : DataTypeConversion
  Divide : Product  Inputs=*/
  Divide1 : Product  Inputs=*/
  Divide2 : Product  Inputs=*/
  Floor : Rounding
  Floor1 : Rounding
  Floor2 : Rounding
  SigOut : Outport
  wires:
  Task_Time_s/1 -> [TaskTime_s]
  Chart/1(out) -> SigOut/1
  Wait_s/1 -> [Wait_s]
  Cycle_cnt/1 -> [Cycle_cnt]
  [OFF_s] -> Divide1/1  "OFF_s"
  [ON_s] -> Divide/1  "ON_s"
  [TaskTime_s] -> Divide1/2
  [Wait_s] -> Divide2/1  "Wait_s"
  [TaskTime_s] -> Divide2/2
  [TaskTime_s] -> Divide/2
  OFF_s/1 -> [OFF_s]
  ON_s/1 -> [ON_s]
  [Cycle_cnt] -> Add/1  "Cycle_cnt"
  Constant4/1 -> Add/2
  Divide2/1 -> Floor2/1
  Divide1/1 -> Floor1/1
  Divide/1 -> Floor/1
  Data Type Conversion1/1 -> Chart/4(Cycle_cnt)
  Data Type Conversion2/1 -> Chart/2(OFF_cnt)
  Data Type Conversion3/1 -> Chart/3(WAIT_cnt)
  Floor1/1 -> Data Type Conversion2/1  "OFF_cnt"
  Floor/1 -> Data Type Conversion/1  "ON_cnt"
  Floor2/1 -> Data Type Conversion3/1  "WAIT_cnt"
  Add/1 -> Data Type Conversion1/1  "Cycle_cnt"
  Data Type Conversion/1 -> Chart/1(ON_cnt)

== system pmm/PMM/PowerModeManagement/PMM Flag Creator /Low Battery Voltage/Low Voltage Charge Pre-Action Flasher/Reverse Buzzer Flasher ==
  Task_Time_s : Inport
  ON_s : Inport  Port=2
  OFF_s : Inport  Port=3
  Cycle_cnt : Inport  Port=4
  Wait_s : Inport  Port=5
  Add : Sum  Inputs=+-
  Chart : Stateflow chart  TreatAsAtomicUnit=on
  Constant4 : Constant  Value=ONE_INT
  Data Type Conversion{,1..3} (4 alike) : DataTypeConversion
  Divide : Product  Inputs=*/
  Divide1 : Product  Inputs=*/
  Divide2 : Product  Inputs=*/
  Floor : Rounding
  Floor1 : Rounding
  Floor2 : Rounding
  SigOut : Outport
  wires:
  Task_Time_s/1 -> [TaskTime_s]
  Wait_s/1 -> [Wait_s]
  Cycle_cnt/1 -> [Cycle_cnt]
  [OFF_s] -> Divide1/1  "OFF_s"
  [ON_s] -> Divide/1  "ON_s"
  [TaskTime_s] -> Divide1/2
  [Wait_s] -> Divide2/1  "Wait_s"
  [TaskTime_s] -> Divide2/2
  [TaskTime_s] -> Divide/2
  OFF_s/1 -> [OFF_s]
  ON_s/1 -> [ON_s]
  [Cycle_cnt] -> Add/1  "Cycle_cnt"
  Constant4/1 -> Add/2
  Divide2/1 -> Floor2/1
  Divide1/1 -> Floor1/1
  Divide/1 -> Floor/1
  Data Type Conversion1/1 -> Chart/4(Cycle_cnt)
  Data Type Conversion2/1 -> Chart/2(OFF_cnt)
  Data Type Conversion3/1 -> Chart/3(WAIT_cnt)
  Floor1/1 -> Data Type Conversion2/1  "OFF_cnt"
  Floor/1 -> Data Type Conversion/1  "ON_cnt"
  Floor2/1 -> Data Type Conversion3/1  "WAIT_cnt"
  Add/1 -> Data Type Conversion1/1  "Cycle_cnt"
  Data Type Conversion/1 -> Chart/1(ON_cnt)
  Chart/1(out) -> SigOut/1

== system pmm/PMM/PowerModeManagement/PMM Flag Creator /Low Battery Voltage/Low Voltage Charge Pre-Action Flasher/Reverse Lamp Flasher ==
  Task_Time_s : Inport
  ON_s : Inport  Port=2
  OFF_s : Inport  Port=3
  Cycle_cnt : Inport  Port=4
  Wait_s : Inport  Port=5
  Add : Sum  Inputs=+-
  Chart : Stateflow chart  TreatAsAtomicUnit=on
  Constant4 : Constant  Value=ONE_INT
  Data Type Conversion{,1..3} (4 alike) : DataTypeConversion
  Divide : Product  Inputs=*/
  Divide1 : Product  Inputs=*/
  Divide2 : Product  Inputs=*/
  Floor : Rounding
  Floor1 : Rounding
  Floor2 : Rounding
  SigOut : Outport
  wires:
  Divide/1 -> Floor/1
  Divide1/1 -> Floor1/1
  Divide2/1 -> Floor2/1
  Constant4/1 -> Add/2
  [Cycle_cnt] -> Add/1  "Cycle_cnt"
  ON_s/1 -> [ON_s]
  OFF_s/1 -> [OFF_s]
  [TaskTime_s] -> Divide/2
  [TaskTime_s] -> Divide2/2
  [Wait_s] -> Divide2/1  "Wait_s"
  [TaskTime_s] -> Divide1/2
  [ON_s] -> Divide/1  "ON_s"
  [OFF_s] -> Divide1/1  "OFF_s"
  Cycle_cnt/1 -> [Cycle_cnt]
  Wait_s/1 -> [Wait_s]
  Chart/1(out) -> SigOut/1
  Task_Time_s/1 -> [TaskTime_s]
  Data Type Conversion1/1 -> Chart/4(Cycle_cnt)
  Data Type Conversion2/1 -> Chart/2(OFF_cnt)
  Data Type Conversion3/1 -> Chart/3(WAIT_cnt)
  Floor1/1 -> Data Type Conversion2/1  "OFF_cnt"
  Floor/1 -> Data Type Conversion/1  "ON_cnt"
  Floor2/1 -> Data Type Conversion3/1  "WAIT_cnt"
  Add/1 -> Data Type Conversion1/1  "Cycle_cnt"
  Data Type Conversion/1 -> Chart/1(ON_cnt)

== stateflow chart pmm/PMM/PowerModeManagement/PMM Flag Creator /Low Battery Voltage/Low Voltage Charge Pre-Action Flasher/Reverse Buzzer Flasher/Chart ==
  state init
    en:
    time_cnt = 0;
    ON_flg = TRUE;
    OFF_flg = FALSE;
    out = 0;
    CycleCnt_cnt = 0;
  state OFF
    en:
    out = 0;
    time_cnt = 0;
    OFF -> (junction 38) [order 1]
    (junction 38) -> OFF : {time_cnt = time_cnt + 1;}
  state ON
    en:
    out = 1;
    time_cnt = 0;
    du:
    time_cnt = time_cnt +1;
  state WAIT
    en:
    out = 0;
    time_cnt = 0;
    du:
    time_cnt = time_cnt + 1;
  (default) -> init
  init -> (junction 57)
  (junction 57) -> ON : [ON_flg]
  OFF -> (junction 46) [order 2] : [time_cnt > OFF_cnt]
  (junction 46) -> (junction 47) : {time_cnt = 0; ON_flg = TRUE; OFF_flg = FALSE; CycleCnt_cnt = CycleCnt_cnt +1;}
  (junction 47) -> ON : [ON_flg]
  ON -> (junction 44) : [time_cnt > ON_cnt]
  (junction 44) -> (junction 42) : {time_cnt = 0; ON_flg = FALSE; OFF_flg = TRUE;}
  (junction 42) -> OFF : [OFF_flg]
  OFF -> (junction 66) [order 1] : [time_cnt > OFF_cnt && CycleCnt_cnt >= Cycle_cnt]
  (junction 66) -> WAIT : {time_cnt = 0;}
  (junction 62) -> ON : {time_cnt = 0; ON_flg = TRUE; OFF_flg = FALSE; CycleCnt_cnt = 0;}
  WAIT -> (junction 62) : [time_cnt >= WAIT_cnt]
  data: ON_cnt input uint32; OFF_cnt input uint32; WAIT_cnt input uint32; Cycle_cnt input uint32; out output uint8; time_cnt local uint32; OFF_flg local boolean; ON_flg local boolean; CycleCnt_cnt local uint32; FALSE parameter; TRUE parameter

== stateflow chart pmm/PMM/PowerModeManagement/PMM Switch Enum Creator/ChrgFault_SW/Subsystem/Chart ==
  state sw
    en:
    a_flg = 0 ;
    b_flg = 0;
    c_flg = 0;
    d_flg = 0;
    e_flg = 0;
    f_flg = 0;
    g_flg = 0;
    h_flg = 0;
    i_flg = 0;
    du:
    cnt = a_in+b_in+c_in+d_in+e_in+f_in+g_in+h_in+i_in;
    (default) -> (junction 156)
    sw -> (junction 156)
    (junction 156) -> (junction 170) [order 1] : [a_in == 1 && a_flg == 0]
    (junction 156) -> (junction 162) [order 2]
    (junction 170) -> (junction 155) : {OUT_ = a_enum;
        | a_flg =1;
        | cnt1 = cnt1 + 1;}
    (junction 162) -> (junction 160) [order 1] : [b_in == 1 && b_flg == 0]
    (junction 162) -> (junction 169) [order 2]
    (junction 160) -> (junction 153) : {OUT_ = b_enum;
        | b_flg =1;
        | cnt1 = cnt1 + 1;}
    (junction 169) -> (junction 171) [order 1] : [c_in == 1 && c_flg == 0]
    (junction 169) -> (junction 177) [order 2]
    (junction 171) -> (junction 168) : {OUT_ = c_enum;
        | c_flg =1;
        | cnt1 = cnt1 + 1;}
    (junction 177) -> (junction 166) [order 1] : [d_in == 1 && d_flg == 0]
    (junction 177) -> (junction 161) [order 2]
    (junction 166) -> (junction 154) : {OUT_ = d_enum;
        | d_flg =1;
        | cnt1 = cnt1 + 1;}
    (junction 161) -> (junction 163) [order 1] : [e_in == 1 && e_flg == 0]
    (junction 161) -> (junction 150) [order 2]
    (junction 163) -> (junction 149) : {OUT_ = e_enum;
        | e_flg =1;
        | cnt1 = cnt1 + 1;}
    (junction 150) -> (junction 148) [order 1] : [f_in == 1 && f_flg == 0]
    (junction 150) -> (junction 158) [order 2]
    (junction 148) -> (junction 151) : {OUT_ = f_enum;
        | f_flg =1;
        | cnt1 = cnt1 + 1;}
    (junction 158) -> (junction 152) [order 1] : [g_in == 1 && g_flg == 0]
    (junction 158) -> (junction 157) [order 2]
    (junction 152) -> (junction 159) : {OUT_ = g_enum;
        | g_flg =1;
        | cnt1 = cnt1 + 1;}
    (junction 157) -> (junction 135) [order 1] : [h_in == 1 && h_flg == 0]
    (junction 157) -> (junction 167) [order 2]
    (junction 135) -> (junction 165) : {OUT_ = h_enum;
        | h_flg =1;
        | cnt1 = cnt1 + 1;}
    (junction 167) -> (junction 131) [order 1] : [i_in == 1 && i_flg == 0]
    (junction 167) -> (junction 126) [order 2]
    (junction 131) -> (junction 203) : {OUT_ = i_enum;
        | i_flg =1;
        | cnt1 = cnt1 + 1;}
    (junction 126) -> (junction 185) [order 2] : [cnt == cnt1]
    (junction 126) -> (junction 125) [order 1] : [cnt == 0]
    (junction 185) -> (junction 187) : {
        | a_flg = 0 ;
        | b_flg = 0;
        | c_flg = 0;
        | d_flg = 0;
        | e_flg = 0;
        | f_flg = 0;
        | g_flg = 0;
        | h_flg = 0;
        | i_flg = 0;
        | cnt1 = 0;
        | }
    (junction 126) -> (junction 202) [order 3] : {cnt1 = cnt;}
    (junction 125) -> (junction 181) : {OUT_ = 0}
  (default) -> sw
  data: a_in input boolean; b_in input boolean; c_in input boolean; OUT_ output; a_flg local boolean size=1; b_flg local boolean size=1; c_flg local boolean size=1; d_in input boolean; d_flg local boolean size=1; e_in input boolean; f_in input boolean; g_in input boolean; h_in input boolean; i_in input boolean; a_enum input; b_enum input; c_enum input; d_enum input; e_enum input; e_flg local boolean size=1; cnt local uint8 size=1; f_enum input; g_enum input; h_enum input; i_enum input; f_flg local boolean size=1; g_flg local boolean size=1; h_flg local boolean size=1; i_flg local boolean size=1; cnt1 local uint8

== stateflow chart pmm/PMM/PowerModeManagement/PMM Flag Creator /Low Battery Voltage/Low Voltage Charge Pre-Action Flasher/Reverse Lamp Flasher/Chart ==
  state init
    en:
    time_cnt = 0;
    ON_flg = TRUE;
    OFF_flg = FALSE;
    out = 0;
    CycleCnt_cnt = 0;
  state OFF
    en:
    out = 0;
    time_cnt = 0;
    OFF -> (junction 38) [order 1]
    (junction 38) -> OFF : {time_cnt = time_cnt + 1;}
  state ON
    en:
    out = 1;
    time_cnt = 0;
    du:
    time_cnt = time_cnt +1;
  state WAIT
    en:
    out = 0;
    time_cnt = 0;
    du:
    time_cnt = time_cnt + 1;
  (default) -> init
  init -> (junction 57)
  (junction 57) -> ON : [ON_flg]
  OFF -> (junction 46) [order 2] : [time_cnt > OFF_cnt]
  (junction 46) -> (junction 47) : {time_cnt = 0; ON_flg = TRUE; OFF_flg = FALSE; CycleCnt_cnt = CycleCnt_cnt +1;}
  (junction 47) -> ON : [ON_flg]
  ON -> (junction 44) : [time_cnt > ON_cnt]
  (junction 44) -> (junction 42) : {time_cnt = 0; ON_flg = FALSE; OFF_flg = TRUE;}
  (junction 42) -> OFF : [OFF_flg]
  OFF -> (junction 66) [order 1] : [time_cnt > OFF_cnt && CycleCnt_cnt >= Cycle_cnt]
  (junction 66) -> WAIT : {time_cnt = 0;}
  (junction 62) -> ON : {time_cnt = 0; ON_flg = TRUE; OFF_flg = FALSE; CycleCnt_cnt = 0;}
  WAIT -> (junction 62) : [time_cnt >= WAIT_cnt]
  data: ON_cnt input uint32; OFF_cnt input uint32; WAIT_cnt input uint32; Cycle_cnt input uint32; out output uint8; time_cnt local uint32; OFF_flg local boolean; ON_flg local boolean; CycleCnt_cnt local uint32; FALSE parameter; TRUE parameter

== stateflow chart pmm/PMM/PowerModeManagement/PMM Flag Creator /Low Battery Voltage/Low Voltage Charge Pre-Action Flasher/Brake Lamp  Flasher/Chart ==
  state init
    en:
    time_cnt = 0;
    ON_flg = TRUE;
    OFF_flg = FALSE;
    out = 0;
    CycleCnt_cnt = 0;
  state OFF
    en:
    out = 0;
    time_cnt = 0;
    OFF -> (junction 38) [order 1]
    (junction 38) -> OFF : {time_cnt = time_cnt + 1;}
  state ON
    en:
    out = 1;
    time_cnt = 0;
    du:
    time_cnt = time_cnt +1;
  state WAIT
    en:
    out = 0;
    time_cnt = 0;
    du:
    time_cnt = time_cnt + 1;
  (default) -> init
  init -> (junction 57)
  (junction 57) -> ON : [ON_flg]
  OFF -> (junction 46) [order 2] : [time_cnt > OFF_cnt]
  (junction 46) -> (junction 47) : {time_cnt = 0; ON_flg = TRUE; OFF_flg = FALSE; CycleCnt_cnt = CycleCnt_cnt +1;}
  (junction 47) -> ON : [ON_flg]
  ON -> (junction 44) : [time_cnt > ON_cnt]
  (junction 44) -> (junction 42) : {time_cnt = 0; ON_flg = FALSE; OFF_flg = TRUE;}
  (junction 42) -> OFF : [OFF_flg]
  OFF -> (junction 66) [order 1] : [time_cnt > OFF_cnt && CycleCnt_cnt >= Cycle_cnt]
  (junction 66) -> WAIT : {time_cnt = 0;}
  (junction 62) -> ON : {time_cnt = 0; ON_flg = TRUE; OFF_flg = FALSE; CycleCnt_cnt = 0;}
  WAIT -> (junction 62) : [time_cnt >= WAIT_cnt]
  data: ON_cnt input uint32; OFF_cnt input uint32; WAIT_cnt input uint32; Cycle_cnt input uint32; out output uint8; time_cnt local uint32; OFF_flg local boolean; ON_flg local boolean; CycleCnt_cnt local uint32; FALSE parameter; TRUE parameter
